simulink model "Node_N_3D"  (R2024b)
settings: Solver=ode1  StartTime=0.0  StopTime=10.0  FixedStep=0.5e-3  RelTol=1e-3
model workspace (MAT data in the model file):
  cfg.BCL = 0.814
  cfg.SD = 0.002
  cfg.f1 = 0.1
  cfg.f2 = 0.25
  cfg.sigma1sq = 0.0035
  cfg.sigma2sq = 0.007
  cfg.d2 = 1281
  cfg.ERP = 0.1615
  cfg.d0 = -773.2
  cfg.MDP = -85.3
  cfg.VT = 23.81
  cfg.VR = 47.94
  cfg.Vh = -4
  cfg.hr = 0.1
  cfg.hs = 35
  cfg.s = 5
  cfg.j = 0
  cfg.m = 1
  cfg.h = 0.2
  cfg.f = 0.1
  cfg.r = 0.5
  cfg_test = Simulink.Parameter
  cfg_test.Value.BCL = 0.814
  cfg_test.Value.SD = 0.002
  cfg_test.Value.f1 = 0.1
  cfg_test.Value.f2 = 0.25
  cfg_test.Value.sigma1sq = 0.0035
  cfg_test.Value.sigma2sq = 0.007
  cfg_test.Value.d2 = 1281
  cfg_test.Value.ERP = 0.1615
  cfg_test.Value.d0 = -773.2
  cfg_test.Value.MDP = -85.3
  cfg_test.Value.VT = 23.81
  cfg_test.Value.VR = 47.94
  cfg_test.Value.Vh = -4
  cfg_test.Value.hr = 0.1
  cfg_test.Value.hs = 35
  cfg_test.Value.s = 5
  cfg_test.Value.j = 0
  cfg_test.Value.m = 1
  cfg_test.Value.h = 0.2
  cfg_test.Value.f = 0.1
  cfg_test.Value.r = 0.5
  cfg_test.Complexity = 'real'
  cfg_test.Dimensions = [1 1]
  cfg_test.DataType = 'Bus: Config_N'
settings Model: DataDictionary=N_dd.sldd  EnableAccessToBaseWorkspace=off  ParameterArgumentNames=cfg_test  Creator=wai484  LastModifiedBy=wai484
settings SolverCC: EnableFixedStepZeroCrossing=on
settings OptimizationCC: UseDivisionForNetSlopeComputation=UseDivisionForReciprocalsOfIntegersOnly

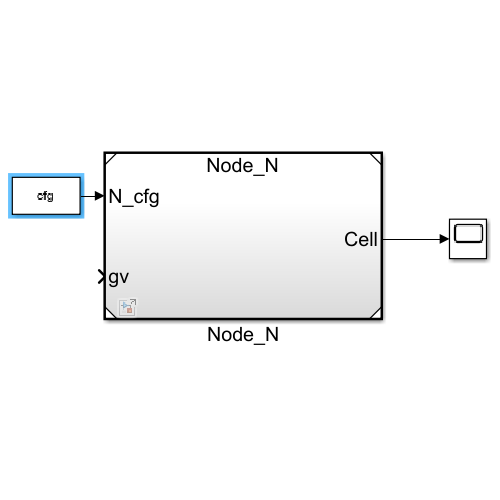
[thumbnail: Simulink's stored preview of the top-level diagram]
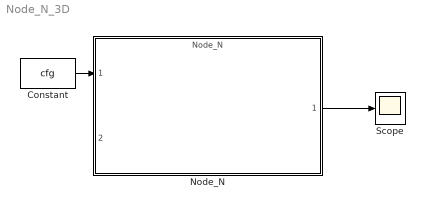
== system Node_N_3D ==
  Constant : Constant  Value=cfg  OutDataTypeStr=Bus: Config_N  SampleTime=-1
  Node_N : ModelReference  ModelNameDialog=Node_N  SimulationMode=Normal  ModelReferenceVersion=1.106
  Scope : Scope
  wires:
  Constant/1 -> Node_N/1
  Node_N/1 -> Scope/1
